simulink model "EEE3099S_Group12_Maze_Sim"  (R2022a)
settings: Solver=FixedStepDiscrete  StartTime=0.0  StopTime=10  FixedStep=0.01  RelTol=1e-3  EnableMultiTasking=on
values from neighbouring files (symbols this model uses):
  axleLength = 0.136    [robotParameters.m]
  ticksPerRot = 20    [robotParameters.m]
  wheelR = 0.031    [robotParameters.m]
undefined symbols (not defined in the file or in its folder): InputPWM, WheelSpeed
libraries: arduinolib x11, spsEdgeDetectorLib x2, slpidlib x1, simulink_extras x1, mobileRoboticsTrainingLib x1
settings Model: ExtModeTrigDuration=2  Creator=Boitumelo  LastModifiedBy=seanpoole
settings SolverCC: AutoInsertRateTranBlk=on
settings OptimizationCC: EnhancedBackFolding=on  PassReuseOutputArgsThreshold=0  MaxStackSize=64  OptimizeBlockOrder=speed  DifferentSizesBufferReuse=on  OptimizationCustomize=off
settings DebuggingCC: MultiTaskDSMMsg=none  ParameterTunabilityLossMsg=error  UnconnectedInputMsg=warning  UnconnectedOutputMsg=warning  UnconnectedLineMsg=warning
settings HardwareCC: ProdBitPerInt=16  ProdBitPerPointer=16  ProdBitPerSizeT=16  ProdBitPerPtrDiffT=16  ProdLargestAtomicFloat=None  ProdWordSize=8  ProdHWDeviceType=Atmel->AVR  UseEmbeddedCoderFeatures=off  UseSimulinkCoderFeatures=off
settings SFSimCC: MATLABDynamicMemAlloc=off
settings RTWCC: SystemTargetFile=ert.tlc  HardwareBoard=Arduino Leonardo  TemplateMakefile=ert_default_tmf  Toolchain=Arduino AVR  BuildConfiguration=Faster Runs  DLArmComputeVersion=19.05
settings CodeAppCC: ForceParamTrailComments=on  OperatorAnnotations=on
settings ERTTargetCC: ERTCustomFileBanners=off  SupportContinuousTime=on  SupportNonInlinedSFcns=on  RemoveResetFunc=off  SupportVariableSizeSignals=on  ModelStepFunctionPrototypeControlCompliant=off  ExtModeTransport=3  ExtModeStaticAlloc=on  ExtModeStaticAllocSize=250  ExtModeMexFile=ext_xcp  ExtModeIntrfLevel=Level2 - Open

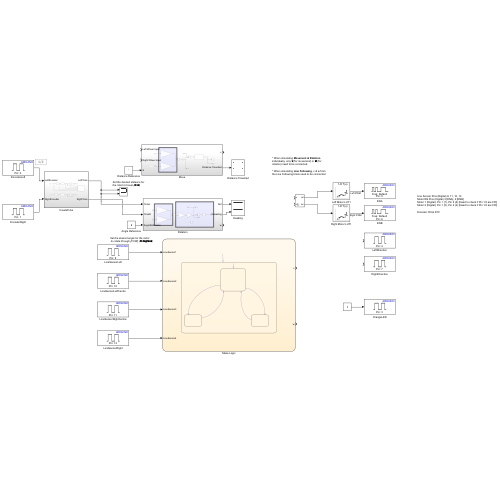
[thumbnail: Simulink's stored preview of the top-level diagram]
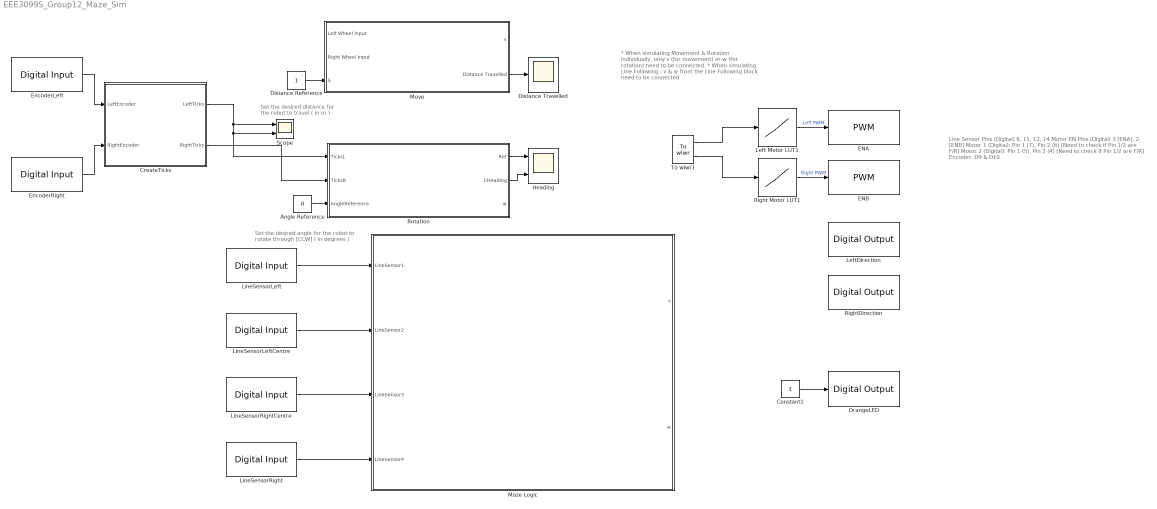
== system EEE3099S_Group12_Maze_Sim ==
  note: Line Sensor Pins (Digital) 8, 11, 12, 14
      | Motor EN Pins (Digital) 3 [ENA], 2 [ENB]
      | Motor 1 (Digital): Pin 1 (7), Pin 2 (6) [Need to check if Pin 1/2 are F/R]
      | Motor 2 (Digital): Pin 1 (5), Pin 2 (4) [Need to check if Pin 1/2 are F/R]
      |
      | Encoder: D9 & D10
  note: * When simulating Movement & Rotation individually, only v (for movement) or w (for rotation) need to be connected.
      |
      | * When simulating Line Following , v & w from the Line Following block need to be connected
  note: Set the desired distance for
      | the robot to travel ( in m )
  note: Set the desired angle for the robot
      | to rotate through [CCW] ( in degrees )
  Angle Reference : Constant  Value=0
  Constant1 : Constant
  CreateTicks : Subsystem
  Distance Reference : Constant
  Distance Travelled : Scope
  ENA : arduinolib/PWM  pinNumber=5  frequencyType=Default  desiredFrequency=490.2  achievableFrequency=490.2
  ENB : arduinolib/PWM  pinNumber=6  frequencyType=Default  desiredFrequency=490.2  achievableFrequency=490.2
  EncoderLeft : arduinolib/Digital Input  pinNumber=0  mode=Default  Direction=input  SampleTime=0.1  blockPlatform=arduino
  EncoderRight : arduinolib/Digital Input  pinNumber=1  mode=Default  Direction=input  SampleTime=0.1  blockPlatform=arduino
  Heading : Scope  NumInputPorts=2
  Left Motor LUT1 : Lookup_n-D  NumberOfTableDimensions=1  BreakpointsForDimension1=WheelSpeed  Table=InputPWM  InterpMethod=Nearest  ExtrapMethod=Clip  InternalRulePriority=Speed  RndMeth=Simplest
  LeftDirection : arduinolib/Digital Output  pinNumber=4  Direction=output  blockPlatform=arduino
  LineSensorLeft : arduinolib/Digital Input  pinNumber=9  mode=Default  Direction=input  SampleTime=0.1  blockPlatform=arduino
  LineSensorLeftCentre : arduinolib/Digital Input  pinNumber=10  mode=Default  Direction=input  SampleTime=0.1  blockPlatform=arduino
  LineSensorRight : arduinolib/Digital Input  pinNumber=12  mode=Default  Direction=input  SampleTime=0.1  blockPlatform=arduino
  LineSensorRightCentre : arduinolib/Digital Input  pinNumber=11  mode=Default  Direction=input  SampleTime=0.1  blockPlatform=arduino
  Maze Logic : Stateflow chart  TreatAsAtomicUnit=on
  Move : Subsystem
  OrangeLED : arduinolib/Digital Output  pinNumber=3  Direction=output  blockPlatform=arduino
  Right Motor LUT1 : Lookup_n-D  NumberOfTableDimensions=1  BreakpointsForDimension1=WheelSpeed  Table=InputPWM  InterpMethod=Nearest  ExtrapMethod=Clip  InternalRulePriority=Speed  RndMeth=Simplest
  RightDirection : arduinolib/Digital Output  pinNumber=7  Direction=output  blockPlatform=arduino
  Rotation : Subsystem
  Scope : Scope  NumInputPorts=2
  To wlwr1 : mobileRoboticsTrainingLib/To wlwr  axleLength=0.1  wheelR=0.05
  wires:
  Rotation/1(Ref) -> Heading/1
  Rotation/2(CHeading) -> Heading/2
  Angle Reference/1 -> Rotation/3(AngleReference)
  Right Motor LUT1/1 -> ENB/1  "Right PWM"
  To wlwr1/1 -> Left Motor LUT1/1
  To wlwr1/2 -> Right Motor LUT1/1
  Left Motor LUT1/1 -> ENA/1  "Left PWM"
  Move/2(Distance Travelled) -> Distance Travelled/1
  Distance Reference/1 -> Move/3(S)
  LineSensorLeft/1 -> Maze Logic/1(LineSensor1)
  LineSensorLeftCentre/1 -> Maze Logic/2(LineSensor2)
  EncoderRight/1 -> CreateTicks/2(RightEncoder)
  EncoderLeft/1 -> CreateTicks/1(LeftEncoder)
  CreateTicks/1(LeftTicks) -> Scope/1, Rotation/1(TicksL), Scope/2
  CreateTicks/2(RightTicks) -> Rotation/2(TicksR)
  Constant1/1 -> OrangeLED/1
  LineSensorRight/1 -> Maze Logic/4(LineSensor4)
  LineSensorRightCentre/1 -> Maze Logic/3(LineSensor3)

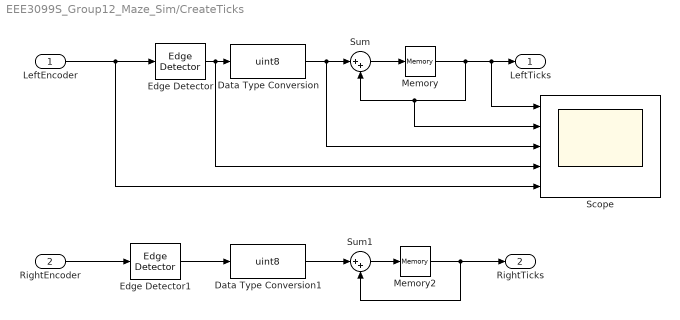
== system EEE3099S_Group12_Maze_Sim/CreateTicks ==
  LeftEncoder : Inport
  RightEncoder : Inport  Port=2
  Data Type Conversion : DataTypeConversion  OutDataTypeStr=uint8  SaturateOnIntegerOverflow=off  RndMeth=Floor
  Data Type Conversion1 : DataTypeConversion  OutDataTypeStr=uint8  SaturateOnIntegerOverflow=off  RndMeth=Floor
  Edge Detector : spsEdgeDetectorLib/Edge Detector  model=Rising  ic=0  Ts=0
      settings: SourceProductBaseCode=PS
  Edge Detector1 : spsEdgeDetectorLib/Edge Detector  model=Rising  ic=0  Ts=0
      settings: SourceProductBaseCode=PS
  Memory : Memory
  Memory2 : Memory
  Scope : Scope  NumInputPorts=5
  Sum : Sum  Inputs=|++
  Sum1 : Sum  Inputs=|++
  LeftTicks : Outport
  RightTicks : Outport  Port=2
  wires:
  Edge Detector1/1 -> Data Type Conversion1/1
  RightEncoder/1 -> Edge Detector1/1
  Edge Detector/1 -> Scope/4, Data Type Conversion/1
  Memory/1 -> Scope/2, Sum/2, Scope/1, LeftTicks/1
  Sum/1 -> Memory/1
  Sum1/1 -> Memory2/1
  Data Type Conversion1/1 -> Sum1/1
  LeftEncoder/1 -> Scope/5, Edge Detector/1
  Memory2/1 -> Sum1/2, RightTicks/1
  Data Type Conversion/1 -> Scope/3, Sum/1

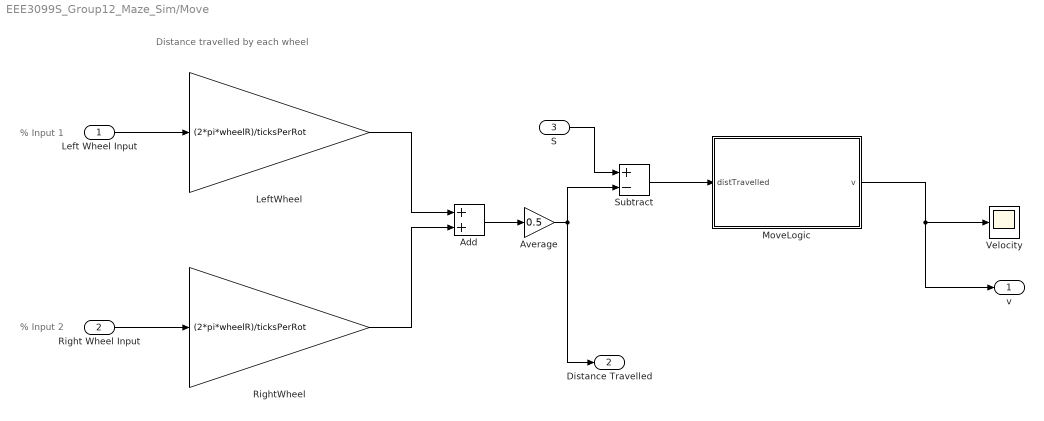
== system EEE3099S_Group12_Maze_Sim/Move ==
  note: Distance travelled by each wheel
  note: % Input 1
  note: % Input 2
  Left Wheel Input : Inport
  Right Wheel Input : Inport  Port=2
  S : Inport  Port=3
  Add : Sum
  Average : Gain  Gain=0.5
  LeftWheel : Gain  Gain=(2*pi*wheelR)/ticksPerRot
  MoveLogic : Stateflow chart  TreatAsAtomicUnit=on
  RightWheel : Gain  Gain=(2*pi*wheelR)/ticksPerRot
  Subtract : Sum  Inputs=+-
  Velocity : Scope
  v : Outport
  Distance Travelled : Outport  Port=2
  wires:
  Left Wheel Input/1 -> LeftWheel/1
  LeftWheel/1 -> Add/1
  Right Wheel Input/1 -> RightWheel/1
  S/1 -> Subtract/1
  RightWheel/1 -> Add/2
  Add/1 -> Average/1
  Average/1 -> Distance Travelled/1, Subtract/2
  Subtract/1 -> MoveLogic/1(distTravelled)
  MoveLogic/1(v) -> v/1, Velocity/1

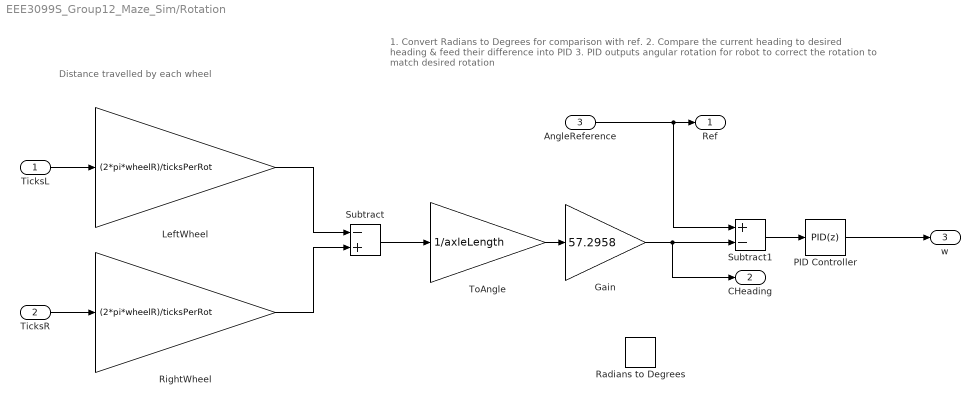
== system EEE3099S_Group12_Maze_Sim/Rotation ==
  note: 1. Convert Radians to Degrees for comparison with ref.
      | 2. Compare the current heading to desired heading
      | & feed their difference into PID
      | 3. PID outputs angular rotation for robot to correct
      | the rotation to match desired rotation
  note: Distance travelled by each wheel
  TicksL : Inport
  TicksR : Inport  Port=2
  AngleReference : Inport  Port=3
  Gain : Gain  Gain=57.2958
  LeftWheel : Gain  Gain=(2*pi*wheelR)/ticksPerRot
  PID Controller : slpidlib/PID Controller  Controller=PID  Form=Parallel  TimeDomain=Discrete-time  UseExternalTs=off  SampleTime=-1  IntegratorMethod=Forward Euler  FilterMethod=Forward Euler  ControllerParametersSource=internal  P=0.111  I=0.001  UseKiTs=off  D=0  N=100  UseFilter=off  TunerSelectOption=Transfer Function Based (PID Tuner App)  InitialConditionSource=internal  InitialConditionForIntegrator=0  InitialConditionForFilter=0  DifferentiatorICPrevScaledInput=0  ExternalReset=none  TrackingMode=off  Kt=1  LimitOutput=on  SatLimitsSource=internal  UpperSaturationLimit=4  LowerSaturationLimit=-4  LinearizeAsGain=on  AntiWindupMode=clamping  Kb=1  POutMin=[]  POutMax=[]  IOutMin=[]  IOutMax=[]  DOutMin=[]  DOutMax=[]  NOutMin=[]  NOutMax=[]  SumOutMin=[]  SumOutMax=[]  SaturationOutMin=[]  SaturationOutMax=[]  PParamMin=[]  PParamMax=[]  IParamMin=[]  IParamMax=[]  DParamMin=[]  DParamMax=[]  NParamMin=[]  NParamMax=[]  KbParamMin=[]  KbParamMax=[]  KtParamMin=[]  KtParamMax=[]  KbOutMin=[]  KbOutMax=[]  KtOutMin=[]  KtOutMax=[]  IntegratorOutMin=[]  IntegratorOutMax=[]  FilterOutMin=[]  FilterOutMax=[]  SumI1OutMin=[]  SumI1OutMax=[]  SumI2OutMin=[]  SumI2OutMax=[]  SumI3OutMin=[]  SumI3OutMax=[]  SumI4OutMin=[]  SumI4OutMax=[]  SumDOutMin=[]  SumDOutMax=[]  DifferentiatorOutMin=[]  DifferentiatorOutMax=[]  FilterDiffOutCoefMin=[]  FilterDiffOutCoefMax=[]  ReciprocalOutMin=[]  ReciprocalOutMax=[]  SumDenOutMin=[]  SumDenOutMax=[]  SumNumOutMin=[]  SumNumOutMax=[]  DivideOutMin=[]  DivideOutMax=[]  UdiffTsProdOutMin=[]  UdiffTsProdOutMax=[]  NTsProdOutMin=[]  NTsProdOutMax=[]  UintegralTsProdOutMin=[]  UintegralTsProdOutMax=[]  UngainTsProdOutMin=[]  UngainTsProdOutMax=[]  IntegratorContinuousStateAttributes=''  IntegratorStateMustResolveToSignalObject=off  IntegratorRTWStateStorageClass=Auto  FilterContinuousStateAttributes=''  FilterStateMustResolveToSignalObject=off  FilterRTWStateStorageClass=Auto  ParallelPVariant=InternalParameters  IdealPVariant=Disabled  IVariant=InternalParameters  DVariant=InternalParameters  IntegratorVariant=Discrete  SatVariant=Enabled  AWVariant=DiscClampingParallel  PCopyVariant=Disabled  TRVariant=Disabled  FdbkBlocksVariant=Forward  IdealPFdbkVariant=Disabled  SatFdbkVariant=Disabled  DerivativeFilterVariant=Differentiator  NVariant=Passthrough  NCopyVariant=Disabled_SignalSpec  FilterICVariant=InternalICsDifferentiator  IntegratorICVariant=InternalICs  ExternalResetVariant=Disabled  TRSumVariant=Passthrough  SumFdbkVariant=Disabled  SumVariant=Sum_PID  TsampFilterVariant=InternalTs  TsampNgainVariant=Passthrough  TsampIntegralVariant=Passthrough  ExternalSaturationOutDataTypeStr=Inherit: Same as second input  aMode=0  InitialConditionSetting=Output
  Radians to Degrees : simulink_extras/Transformations/Radians to Degrees
  RightWheel : Gain  Gain=(2*pi*wheelR)/ticksPerRot
  Subtract : Sum  Inputs=-+
  Subtract1 : Sum  Inputs=+-
  ToAngle : Gain  Gain=1/axleLength
  Ref : Outport
  CHeading : Outport  Port=2
  w : Outport  Port=3
  wires:
  RightWheel/1 -> Subtract/2
  LeftWheel/1 -> Subtract/1
  Subtract/1 -> ToAngle/1
  Subtract1/1 -> PID Controller/1
  Gain/1 -> CHeading/1, Subtract1/2
  AngleReference/1 -> Ref/1, Subtract1/1
  TicksL/1 -> LeftWheel/1
  ToAngle/1 -> Gain/1
  TicksR/1 -> RightWheel/1
  PID Controller/1 -> w/1

== stateflow chart EEE3099S_Group12_Maze_Sim/Maze Logic ==
  state CrossRoad
    state MoveBack
      v=0.035;
      dirL = 1;
      dirR = 1;
    (default) -> MoveBack
  state FollowLine
    state Straight
      entry:
      v=0.035;
      w=0;
    note: % If LHS, middle sensor doesn't detect a line, correct this by bearing right
    note: % If RHS, middle sensor doesn't detect a line, correct this by bearing left
    state BearRight
      entry:
      w=-0.2;
    state BearLeft
      entry:
      w=0.2;
    (default) -> Straight
    Straight -> BearRight [order 2] : [LineSensor2<1]
    Straight -> BearLeft [order 1] : [LineSensor3<1]
    BearRight -> Straight : [LineSensor3>=1 && LineSensor2>=1]
    BearLeft -> Straight : [LineSensor3>=1 && LineSensor2>=1]
  state Decision
    v=0.035;
    y=elapsed(sec);
  state EndOfMaze
    v=0;
  state RiverCrossing
    state MoveForward
      v=0.035;
    (default) -> MoveForward
  note: % Both middle sensors detect a line, and the robot can continue going straight
  (default) -> FollowLine : % Idle State
  Decision -> CrossRoad [order 3] : [y>=2 && LineSensor1==0 && LineSensor2==1 && LineSensor3==1 && LineSensor4==0]
  FollowLine -> Decision : [LineSensor1==0 && LineSensor2==0 && LineSensor3==0 && LineSensor4==0]
  Decision -> EndOfMaze [order 2] : [y>=2 && LineSensor1==0 && LineSensor2==0 && LineSensor3==0 && LineSensor4==0]
  Decision -> RiverCrossing [order 1] : [y>=2 && LineSensor1==1 && LineSensor2==1 && LineSensor3==1 && LineSensor4==1]
  RiverCrossing -> FollowLine : [LineSensor2 == 1 && LineSensor3 == 1]
  data: v output; w output; LineSensor1 input; LineSensor2 input; LineSensor3 input; LineSensor4 input

== stateflow chart EEE3099S_Group12_Maze_Sim/Move/MoveLogic ==
  state MoveForward
    entry:
    v=0.1;
  state Stop
    entry:
    v=0;
  (default) -> MoveForward
  MoveForward -> Stop : [distTravelled <= 1]
  data: distTravelled input; v output
